simulink model "stock_stateflow_2013b"  (R2013b)
settings: Solver=ode45  StartTime=0.0  StopTime=10.0  RelTol=1e-3
undefined symbols (not defined in the file): appl, appl_len
settings Model: Creator=pound  LastModifiedBy=pound
settings DebuggingCC: FrameProcessingCompatibilityMsg=error
settings GRTTargetCC: CodeReplacementLibrary=C89/C90 (ANSI)

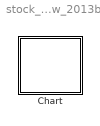
== system stock_stateflow_2013b ==
  Chart : Stateflow chart  TreatAsAtomicUnit=on
      settings: PermitHierarchicalResolution=ParametersOnly

== stateflow chart stock_stateflow_2013b/Chart ==
  state init
  state Fractal_Buy
  state Idle
    L = 0 %Blue
    M = 0  %Red
    S = 0 %Green
    FB = 0
    FS = 1
  state Fractal_Sell
  state Sell
  state Hold
  state Buy
  (default) -> init
  (junction 75) -> Fractal_Buy [order 1] : [S > M && M > L]
  (junction 55) -> (junction 55) [order 1] : [i > appl_len-9]{L = L + appl[i];...
      |           M = M + appl[i];...
      |           i--;}
  (junction 56) -> (junction 75) [order 2] : {S = S/5.0;...
      | M = M/8.0;...
      | L = L/13.0;}
  (junction 55) -> (junction 56) [order 2]
  (junction 53) -> (junction 55) [order 2]
  Idle -> (junction 53) : {i=appl_len-1;}
  (junction 75) -> Fractal_Sell [order 2] : [L > M && M > S]
  (junction 56) -> (junction 56) [order 1] : [i>appl_len-14]{L = L + appl[i]; i--}
  (junction 53) -> (junction 53) [order 1] : [i > appl_len-6]{L = L + appl[i];...
      |         M = M + appl[i];...
      |         S = S + appl[i];...
      |         i--;}
  (junction 75) -> Hold [order 3]
  init -> Idle
  Fractal_Buy -> Hold [order 1] : [!FB]
  Fractal_Buy -> Buy [order 2] : [FB]
  Buy -> Idle
  Hold -> Idle
  Sell -> Idle
  Fractal_Sell -> Sell [order 1] : [FS]
  Fractal_Sell -> Hold [order 2] : [!FS]
  data: FB local double; FS local double; L local double; M local double; S local double; appl parameter double size=appl_len; i local double; sum local double; appl_len parameter
